simulink model "robot_turn"  (R2023a)
settings: Solver=FixedStepDiscrete  StartTime=0.0  StopTime=100  FixedStep=0.01  RelTol=1e-3
libraries: mobileRoboticsTrainingLib x3
settings Model: Creator=Boitumelo  LastModifiedBy=thuto
settings DebuggingCC: UnconnectedInputMsg=warning  UnconnectedOutputMsg=warning  UnconnectedLineMsg=warning
settings ModelReferenceCC: EnableRefExpFcnMdlSchedulingChecks=on
settings RTWCC: DLArmComputeVersion=19.05

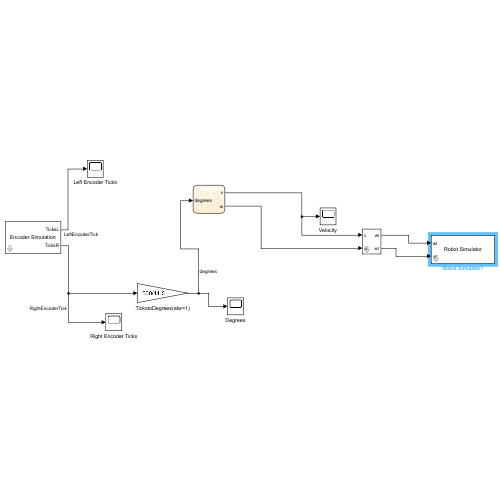
[thumbnail: Simulink's stored preview of the top-level diagram]
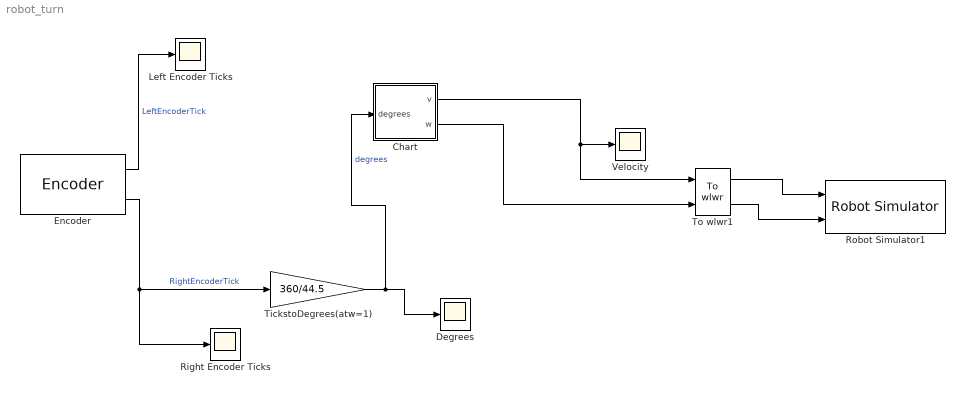
== system robot_turn ==
  Chart : Stateflow chart  TreatAsAtomicUnit=on
  Degrees : Scope
  Encoder : mobileRoboticsTrainingLib/Encoder  axleLength=axleLength  wheelR=wheelR  ticksPerRot=ticksPerRot
      settings: SourceProductName=Mobile Robotics Training Library
  Left Encoder Ticks : Scope
  Right Encoder Ticks : Scope
  Robot Simulator1 : mobileRoboticsTrainingLib/Robot Simulator  Priority=99  mapVar=mapForSim  startX=0.50483  startY=0.10878  startTheta=0  axleLength=axleLength  wheelR=wheelR
  TickstoDegrees(atw=1) : Gain  Gain=360/44.5
  To wlwr1 : mobileRoboticsTrainingLib/To wlwr  axleLength=0.1  wheelR=0.05
  Velocity : Scope
  wires:
  Encoder/1 -> Left Encoder Ticks/1  "LeftEncoderTick"
  Encoder/2 -> Right Encoder Ticks/1, TickstoDegrees(atw=1)/1  "RightEncoderTick"
  Chart/1(v) -> To wlwr1/1, Velocity/1
  To wlwr1/1 -> Robot Simulator1/1
  To wlwr1/2 -> Robot Simulator1/2
  Chart/2(w) -> To wlwr1/2
  TickstoDegrees(atw=1)/1 -> Chart/1(degrees), Degrees/1  "degrees"

== stateflow chart robot_turn/Chart ==
  state startTurn1
    entry: v=0
    w=1
  state resetPos1
    entry: v=0
    w=-1
  state startTurn3
    entry: v=0
    w=1
  state resetPos2
    entry: v=0
    w=-1
  state startTurn2
    entry: v=0
    w=1
  state resetPos3
    entry: v=0
    w=-1
  state resetPos4
    entry: v=0
    w=0
  (default) -> startTurn1
  startTurn1 -> resetPos1 : [degrees>= 90]
  resetPos1 -> startTurn2 : [degrees < 0]
  resetPos2 -> startTurn3 : [degrees < 0]
  startTurn2 -> resetPos2 : [degrees>=180]
  startTurn3 -> resetPos3 : [degrees>=270]
  resetPos3 -> resetPos4 : [degrees < 0]
  data: v output; w output; degrees input
